simulink model "uniones_servo_obs"  (R2024b)
settings: Solver=VariableStepAuto  StartTime=0.0  StopTime=10.0  RelTol=1e-3
values from neighbouring files (symbols this model uses):
  A = [0 1 0 0 ... (first row only)    [code_cte_small.m]    (also in lab1.m)
  Afcc = inv(T) * A * T    [code_cte_small.m]    (also in lab1.m)
  Afco = inv(Q)*A*Q    [code_cte_small.m]    (also in lab1.m)
  B = [0 ... (first row only)    [code_cte_small.m]    (also in lab1.m)
  Bfcc = inv(T) * B    [code_cte_small.m]    (also in lab1.m)
  Bfco = inv(Q) * B    [code_cte_small.m]    (also in lab1.m)
  C = [1 0 0 0]    [code_cte_small.m]    (also in lab1.m)
  Cfcc = C * T    [code_cte_small.m]    (also in lab1.m)
  Cfco = C * Q    [code_cte_small.m]    (also in lab1.m)
  E = [0 ... (first row only)    [code_cte_small.m]    (also in lab1.m)
  Efcc = inv(T)*E    [code_cte_small.m]    (also in lab1.m)
  Efco = inv(Q) * E    [code_cte_small.m]    (also in lab1.m)
  k_obs_F_matriz = inv(matriz_P_f)*k_cachuchita_f'    [code_cte_small.m]    (also in lab1.m)
  k_obs_FCC_matriz = inv(matriz_P)*k_cachuchita'    [code_cte_small.m]    (also in lab1.m)
  k_obs_FCO_matriz = inv(matriz_P_fco)*k_cachuchita_fco'    [code_cte_small.m]    (also in lab1.m)
  KA = [-19.21, 9.68, 4.10, -15.739]    [code_cte_small.m]    (also in lab1.m = [-15.3759, -7.2896182, -45.976447, -15.168131])
  KAfcc = [-29798.327,25528.529, 7395.9961,14.998605]    [code_cte_small.m]    (also in lab1.m)
  KAfco = [-3.2913256, 1568.6046, -768661.08, 376589940.0 ]    [code_cte_small.m]    (also in lab1.m)
  kiA = -24.76    [code_cte_small.m]    (also in lab1.m = -151.09413)
  kiAfcc = [-151.09413]    [code_cte_small.m]    (also in lab1.m)
  kiAfco = [-151.09413]    [code_cte_small.m]    (also in lab1.m)
settings Model: Creator=Usuario  LastModifiedBy=Usuario

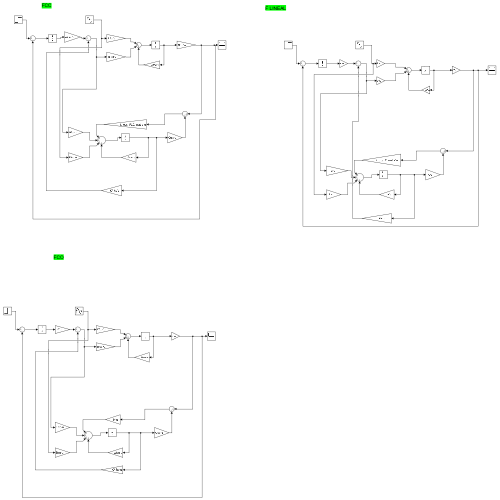
[thumbnail: Simulink's stored preview of the top-level diagram]
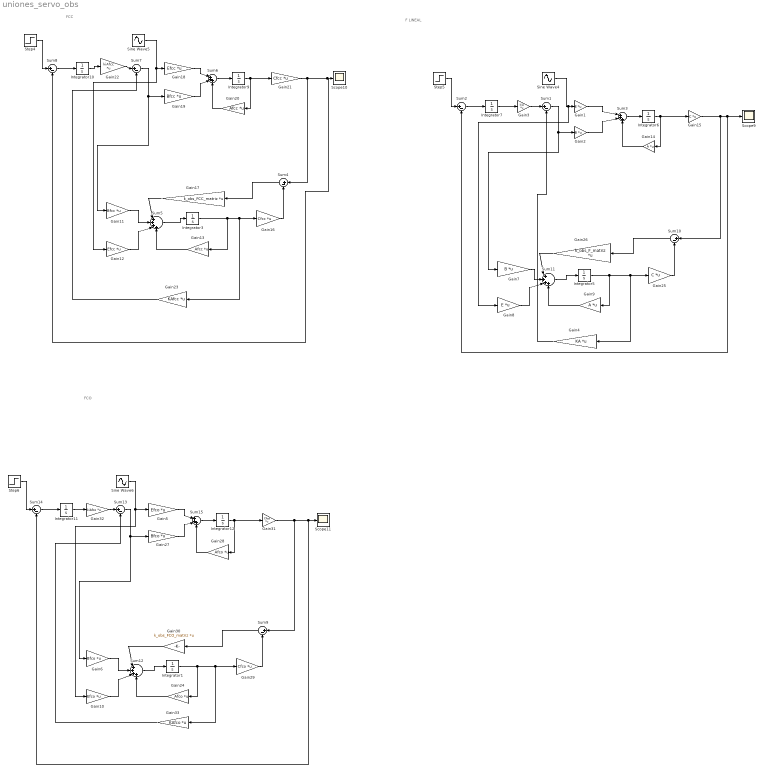
== system uniones_servo_obs ==
  note: F LINEAL
  note: FCC
  note: FCO
  Gain1 : Gain  Gain=E  Multiplication=Matrix(K*u)
  Gain10 : Gain  Gain=Efco  Multiplication=Matrix(K*u)
  Gain11 : Gain  Gain=Bfcc  Multiplication=Matrix(K*u)
  Gain12 : Gain  Gain=Efcc  Multiplication=Matrix(K*u)
  Gain13 : Gain  Gain=Afcc  Multiplication=Matrix(K*u)
  Gain14 : Gain  Gain=A  Multiplication=Matrix(K*u)
  Gain15 : Gain  Gain=C  Multiplication=Matrix(K*u)
  Gain16 : Gain  Gain=Cfcc  Multiplication=Matrix(K*u)
  Gain17 : Gain  Gain=k_obs_FCC_matriz  Multiplication=Matrix(K*u)
  Gain18 : Gain  Gain=Efcc  Multiplication=Matrix(K*u)
  Gain19 : Gain  Gain=Bfcc  Multiplication=Matrix(K*u)
  Gain2 : Gain  Gain=B  Multiplication=Matrix(K*u)
  Gain20 : Gain  Gain=Afcc  Multiplication=Matrix(K*u)
  Gain21 : Gain  Gain=Cfcc  Multiplication=Matrix(K*u)
  Gain22 : Gain  Gain=kiAfcc  Multiplication=Matrix(K*u)
  Gain23 : Gain  Gain=KAfcc  Multiplication=Matrix(K*u)
  Gain24 : Gain  Gain=Afco  Multiplication=Matrix(K*u)
  Gain25 : Gain  Gain=C  Multiplication=Matrix(K*u)
  Gain26 : Gain  Gain=k_obs_F_matriz  Multiplication=Matrix(K*u)
  Gain27 : Gain  Gain=Bfco  Multiplication=Matrix(K*u)
  Gain28 : Gain  Gain=Afco  Multiplication=Matrix(K*u)
  Gain29 : Gain  Gain=Cfco  Multiplication=Matrix(K*u)
  Gain3 : Gain  Gain=kiA  Multiplication=Matrix(K*u)
  Gain30 : Gain  Gain=k_obs_FCO_matriz  Multiplication=Matrix(K*u)
  Gain31 : Gain  Gain=Cfco  Multiplication=Matrix(K*u)
  Gain32 : Gain  Gain=kiAfco  Multiplication=Matrix(K*u)
  Gain33 : Gain  Gain=KAfco  Multiplication=Matrix(K*u)
  Gain4 : Gain  Gain=KA  Multiplication=Matrix(K*u)
  Gain5 : Gain  Gain=Efco  Multiplication=Matrix(K*u)
  Gain6 : Gain  Gain=Bfco  Multiplication=Matrix(K*u)
  Gain7 : Gain  Gain=B  Multiplication=Matrix(K*u)
  Gain8 : Gain  Gain=E  Multiplication=Matrix(K*u)
  Gain9 : Gain  Gain=A  Multiplication=Matrix(K*u)
  Integrator{1,3,5..7,9..12} (9 alike) : Integrator
  Scope10 : Scope
  Scope11 : Scope
  Scope9 : Scope
  Sine Wave4 : Sin  Frequency=5  SampleTime=0
  Sine Wave5 : Sin  Frequency=5  SampleTime=0
  Sine Wave6 : Sin  Frequency=5  SampleTime=0
  Step4 : Step  Time=0  SampleTime=0
  Step5 : Step  Time=0  SampleTime=0
  Step6 : Step  Time=0  SampleTime=0
  Sum{1..2,4,7..10,13..14} (9 alike) : Sum  Inputs=|+-
  Sum11 : Sum  Inputs=|++++
  Sum12 : Sum  Inputs=|++++
  Sum15 : Sum  Inputs=|+++
  Sum3 : Sum  Inputs=|+++
  Sum5 : Sum  Inputs=|++++
  Sum6 : Sum  Inputs=|+++
  wires:
  Step4/1 -> Sum8/1
  Gain18/1 -> Sum6/1
  Integrator9/1 -> Gain20/1, Gain21/1
  Integrator10/1 -> Gain22/1
  Gain19/1 -> Sum6/2
  Gain22/1 -> Sum7/1
  Sum7/1 -> Gain11/1, Gain19/1
  Gain20/1 -> Sum6/3
  Sum8/1 -> Integrator10/1
  Sum6/1 -> Integrator9/1
  Sine Wave5/1 -> Gain12/1, Gain18/1
  Sum5/1 -> Integrator3/1
  Integrator3/1 -> Gain13/1, Gain23/1, Gain16/1
  Sum4/1 -> Gain17/1
  Gain16/1 -> Sum4/2
  Gain11/1 -> Sum5/2
  Gain13/1 -> Sum5/4
  Gain12/1 -> Sum5/3
  Gain17/1 -> Sum5/1
  Gain23/1 -> Sum7/2
  Gain21/1 -> Sum8/2, Scope10/1, Sum4/1
  Step5/1 -> Sum2/1
  Sine Wave4/1 -> Gain8/1, Gain1/1
  Integrator6/1 -> Gain15/1, Gain14/1
  Gain14/1 -> Sum3/3
  Gain2/1 -> Sum3/2
  Gain3/1 -> Sum1/1
  Sum3/1 -> Integrator6/1
  Gain1/1 -> Sum3/1
  Sum2/1 -> Integrator7/1
  Sum1/1 -> Gain7/1, Gain2/1
  Integrator7/1 -> Gain3/1
  Gain8/1 -> Sum11/3
  Integrator5/1 -> Gain9/1, Gain4/1, Gain25/1
  Gain7/1 -> Sum11/2
  Sum11/1 -> Integrator5/1
  Gain25/1 -> Sum10/2
  Sum10/1 -> Gain26/1
  Gain9/1 -> Sum11/4
  Gain26/1 -> Sum11/1
  Gain4/1 -> Sum1/2
  Gain15/1 -> Sum10/1, Sum2/2, Scope9/1
  Gain24/1 -> Sum12/4
  Gain10/1 -> Sum12/3
  Gain29/1 -> Sum9/2
  Sum12/1 -> Integrator1/1
  Gain6/1 -> Sum12/2
  Integrator1/1 -> Gain24/1, Gain33/1, Gain29/1
  Gain30/1 -> Sum12/1
  Sum9/1 -> Gain30/1
  Sum15/1 -> Integrator12/1
  Sum14/1 -> Integrator11/1
  Gain32/1 -> Sum13/1
  Sum13/1 -> Gain6/1, Gain27/1
  Sine Wave6/1 -> Gain10/1, Gain5/1
  Gain5/1 -> Sum15/1
  Gain27/1 -> Sum15/2
  Gain28/1 -> Sum15/3
  Integrator12/1 -> Gain31/1, Gain28/1
  Step6/1 -> Sum14/1
  Integrator11/1 -> Gain32/1
  Gain33/1 -> Sum13/2
  Gain31/1 -> Sum9/1, Sum14/2, Scope11/1
